simulink model "ekstraNul"  (R2015a)
settings: Solver=ode45  StartTime=0.0  StopTime=10  RelTol=1e-3
libraries: cstblocks x10, simulink x5
settings Model: Creator=morten  LastModifiedBy=Steffan

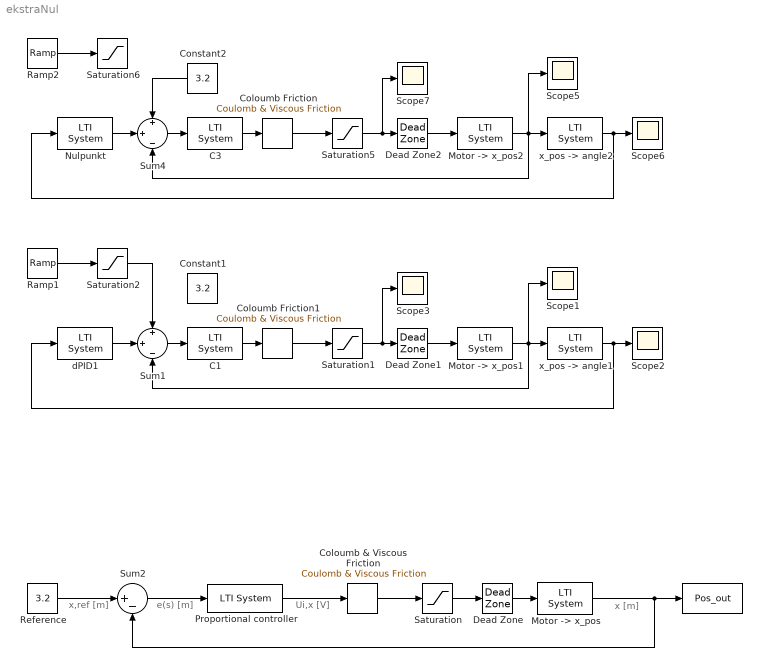
== system ekstraNul ==
  note: x [m]
  note: Ui,x [V]
  note: e(s) [m]
  note: x,ref [m]
  " " : ToWorkspace  VariableName=Pos_out  SaveFormat=Timeseries  SampleTime=-1
  C1 : cstblocks/LTI System  sys=C1  IC=[]
  C3 : cstblocks/LTI System  sys=C1  IC=[]
  Coloumb & Viscous Friction : simulink/Discontinuities/Coulomb & Viscous Friction  offset=[4.2]  gain=1
  Coloumb Friction : simulink/Discontinuities/Coulomb & Viscous Friction  offset=[4.2]  gain=1
  Coloumb Friction1 : simulink/Discontinuities/Coulomb & Viscous Friction  offset=[4.2]  gain=1
  Constant1 : Constant  Value=3.2
  Constant2 : Constant  Value=3.2
  Dead Zone : DeadZone  LowerValue=-4.2  UpperValue=4.2  SaturateOnIntegerOverflow=on
  Dead Zone1 : DeadZone  LowerValue=-4.2  UpperValue=4.2  SaturateOnIntegerOverflow=on
  Dead Zone2 : DeadZone  LowerValue=-4.2  UpperValue=4.2  SaturateOnIntegerOverflow=on
  "Motor -> x_pos" : cstblocks/LTI System  sys=X  IC=[]
  "Motor -> x_pos1" : cstblocks/LTI System  sys=Xm  IC=[]
  "Motor -> x_pos2" : cstblocks/LTI System  sys=Xm  IC=[]
  Nulpunkt : cstblocks/LTI System  sys=dD  IC=[]
  Proportional controller : cstblocks/LTI System  sys=C1  IC=[]
  Ramp1 : simulink/Sources/Ramp  slope=.5  start=0  X0=0
  Ramp2 : simulink/Sources/Ramp  slope=.5  start=0  X0=0
  Reference : Constant  Value=3.2
  Saturation : Saturate  UpperLimit=12.5  LowerLimit=-12.5
  Saturation1 : Saturate  UpperLimit=12.5  LowerLimit=-12.5
  Saturation2 : Saturate  UpperLimit=3.2  LowerLimit=0
  Saturation5 : Saturate  UpperLimit=12.5  LowerLimit=-12.5
  Saturation6 : Saturate  UpperLimit=3.2  LowerLimit=0
  Scope{1..3,5..7} (6 alike) : Scope
      Scope2 settings: YMin=-0.0005  YMax=0.0009
      Scope3 settings: SaveName=ScopeData2
      Scope5 settings: SaveName=ScopeData4
      Scope6 settings: YMin=-0.0005  YMax=0.0009  SaveName=ScopeData5
      Scope7 settings: SaveName=ScopeData6
  Sum1 : Sum  Inputs=+|+|-
  Sum2 : Sum  Inputs=|+-
  Sum4 : Sum  Inputs=+|+|-
  dPID1 : cstblocks/LTI System  sys=k  IC=[]
  "x_pos -> angle1" : cstblocks/LTI System  sys=Wm  IC=[]
  "x_pos -> angle2" : cstblocks/LTI System  sys=Wm  IC=[]
  wires:
  "Motor -> x_pos2"/1 -> Scope5/1, Sum4/3, "x_pos -> angle2"/1
  Saturation5/1 -> Scope7/1, Dead Zone2/1
  Dead Zone2/1 -> "Motor -> x_pos2"/1
  C3/1 -> Coloumb Friction/1
  Constant2/1 -> Sum4/1
  Sum4/1 -> C3/1
  Nulpunkt/1 -> Sum4/2
  Coloumb Friction/1 -> Saturation5/1
  "x_pos -> angle2"/1 -> Nulpunkt/1, Scope6/1
  Ramp2/1 -> Saturation6/1
  "Motor -> x_pos1"/1 -> Scope1/1, Sum1/3, "x_pos -> angle1"/1
  Saturation1/1 -> Scope3/1, Dead Zone1/1
  Dead Zone1/1 -> "Motor -> x_pos1"/1
  C1/1 -> Coloumb Friction1/1
  Saturation2/1 -> Sum1/1
  Sum1/1 -> C1/1
  dPID1/1 -> Sum1/2
  Coloumb Friction1/1 -> Saturation1/1
  "x_pos -> angle1"/1 -> dPID1/1, Scope2/1
  Ramp1/1 -> Saturation2/1
  "Motor -> x_pos"/1 -> " "/1, Sum2/2
  Saturation/1 -> Dead Zone/1
  Dead Zone/1 -> "Motor -> x_pos"/1
  Proportional controller/1 -> Coloumb & Viscous Friction/1
  Sum2/1 -> Proportional controller/1
  Coloumb & Viscous Friction/1 -> Saturation/1
  Reference/1 -> Sum2/1
